simulink model "Design and Analysis of Fuel Cell Vehicle-to-Grid System"  (R2024b)
settings: Solver=VariableStepAuto  StartTime=0.0  StopTime=5  RelTol=1e-3
values from neighbouring files (symbols this model uses):
  Afc = 232.0    (= 232)    [rlpar_1.m]
  F = 96485    [rlpar_1.m]
  K1 = 7.034e-3    (= 0.007034)    [rlpar_1.m]
  K2 = 7.036e-3    (= 0.007036)    [rlpar_1.m]
  N = 35    [rlpar_1.m]
  Pop = 101325    [rlpar_1.m]
  R = 8.314    [rlpar_1.m]
  T = 338.5    [rlpar_1.m]
  Ts = 4e-6    (= 4e-06)    [rlpar_1.m]
  Va = 6.495    [rlpar_1.m]
  YH2 = 0.99    [rlpar_1.m]
  YO2 = 0.21    [rlpar_1.m]
undefined symbols (not defined in the file or in its folder): ln
libraries: powerlib_extras x14, spsSeriesRLCBranchLib x9, spsCurrentMeasurementLib x6, spsIGBTLib x5, spsVoltageMeasurementLib x4, spsControlledVoltageSourceLib x2, spsACVoltageSourceLib x1, spsDCVoltageSourceLib x1, spsDiodeLib x1, spsGroundLib x1, slpidlib x1, spsPWMGeneratorDCDCLib x1
settings Model: Creator=Ashish  LastModifiedBy=Ashish

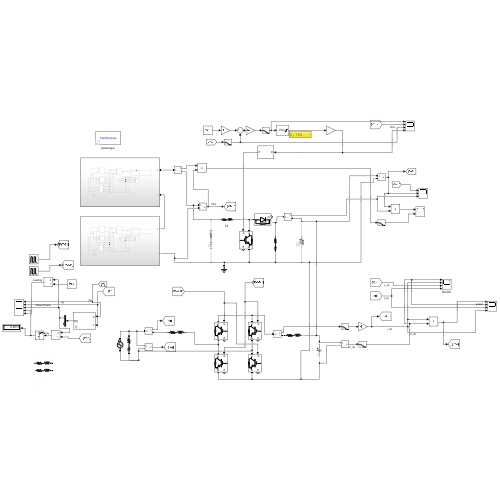
[thumbnail: Simulink's stored preview of the top-level diagram]
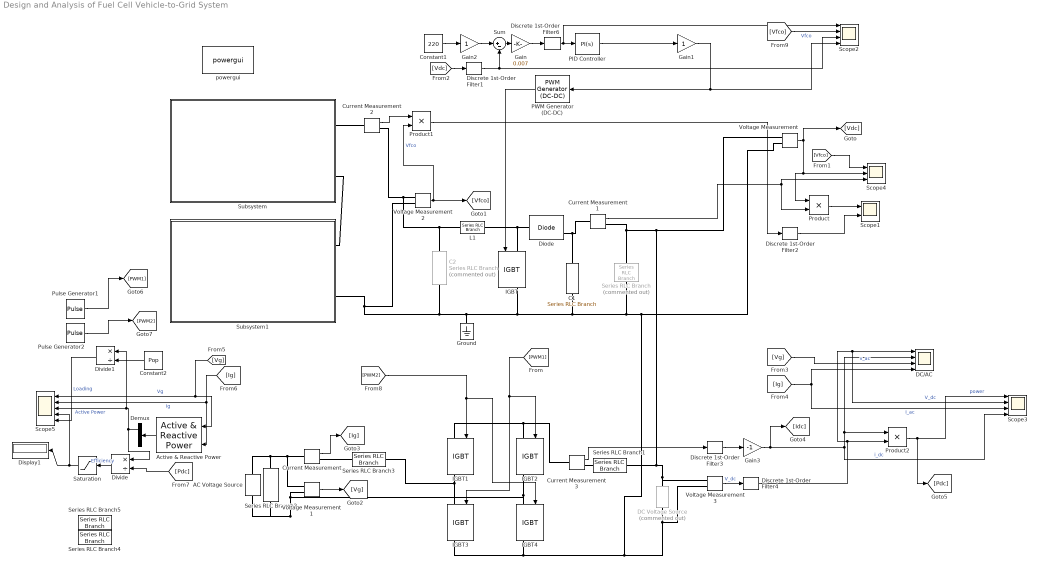
== system Design and Analysis of Fuel Cell Vehicle-to-Grid System ==
  AC Voltage Source : spsACVoltageSourceLib/AC Voltage Source  Amplitude=381  Phase=0  Frequency=50  SampleTime=0  Measurements=None  BusType=swing  Pref=10e3  Qref=0  Qmin=-inf  Qmax=+inf
  Active & Reactive Power : powerlib_extras/Measurements/Active & Reactive Power  f1=50
  C1 : spsSeriesRLCBranchLib/Series RLC Branch  LConnTagsString=__new0  RConnTagsString=__new0  BranchType=RC  Resistance=0.0001  Inductance=1.0  SetiL0=off  InitialCurrent=0  Capacitance=1e-4  Setx0=on  InitialVoltage=0  Measurements=Branch voltage
  C2 : spsSeriesRLCBranchLib/Series RLC Branch  Commented=on  LConnTagsString=__new0  RConnTagsString=__new0  BranchType=RC  Resistance=1.0  Inductance=1.0  SetiL0=off  InitialCurrent=0  Capacitance=1e-1  Setx0=off  InitialVoltage=600  Measurements=Branch voltage
  Constant1 : Constant  Value=220
  Constant2 : Constant  Value=Pop
  Current Measurement{,1..3} (4 alike) : spsCurrentMeasurementLib/Current Measurement  PhasorSimulation=off  OutputType=Complex  PSBequivalent=0
  DC Voltage Source : spsDCVoltageSourceLib/DC Voltage Source  Commented=on  Amplitude=220  Measurements=None
  DC/AC : Scope  NumInputPorts=4
  Demux : Demux  Outputs=2
  Diode : spsDiodeLib/Diode  Ron=0.001  Lon=0  Vf=0.8  IC=0  UseSnubber=off  Rs=500  Cs=250e-9  Measurements=on
  Discrete 1st-Order Filter{1..4,6} (5 alike) : powerlib_extras/Discrete  Control Blocks/Discrete 1st-Order Filter  FilterType=Lowpass  Tc=12e-3  Ts=Ts  Initialize=off  Vac_Init=[0.8 -25 60]  Vdc_Init=-0.4  PlotResponse=off  param1=[1 500 0.1]
  Display1 : Display
  Divide : Product  Inputs=*/
  Divide1 : Product  Inputs=*/
  Gain : Gain  Gain=0.007
  Gain1 : Gain
  Gain2 : Gain
  Gain3 : Gain  Gain=-1
  Ground : spsGroundLib/Ground  LConnTagsString=a
  IGBT{,1..4} (5 alike) : spsIGBTLib/IGBT  Ron=0.001  Lon=0  Vf=1  Tf=1e-6  Tt=2e-6  IC=0  Rs=1e5  Cs=inf  Measurements=on
  L1 : spsSeriesRLCBranchLib/Series RLC Branch  LConnTagsString=__new0  RConnTagsString=__new0  BranchType=RL  Resistance=0.001  Inductance=1e-3  SetiL0=off  InitialCurrent=2  Capacitance=1e-6  Setx0=off  InitialVoltage=0  Measurements=None
  PID Controller : slpidlib/PID Controller  Controller=PI  Form=Parallel  TimeDomain=Continuous-time  UseExternalTs=off  SampleTime=-1  IntegratorMethod=Forward Euler  FilterMethod=Forward Euler  ControllerParametersSource=internal  P=0.6  I=8  UseKiTs=off  D=0  UseExternalDerivativeSource=off  N=100  UseFilter=on  TunerSelectOption=Transfer Function Based (PID Tuner App)  InitialConditionSource=internal  InitialConditionForIntegrator=0.1  InitialConditionForFilter=0  DifferentiatorICPrevScaledInput=0  ExternalReset=none  TrackingMode=off  Kt=1  LimitOutput=on  SatLimitsSource=internal  UpperSaturationLimit=0.99  LowerSaturationLimit=0.1  LinearizeAsGain=on  AntiWindupMode=none  Kb=1  LimitIntegrator=off  UpperIntegratorSaturationLimit=inf  LowerIntegratorSaturationLimit=-inf  POutMin=[]  POutMax=[]  IOutMin=[]  IOutMax=[]  DOutMin=[]  DOutMax=[]  NOutMin=[]  NOutMax=[]  SumOutMin=[]  SumOutMax=[]  SaturationOutMin=[]  SaturationOutMax=[]  PParamMin=[]  PParamMax=[]  IParamMin=[]  IParamMax=[]  DParamMin=[]  DParamMax=[]  NParamMin=[]  NParamMax=[]  KbParamMin=[]  KbParamMax=[]  KtParamMin=[]  KtParamMax=[]  KbOutMin=[]  KbOutMax=[]  KtOutMin=[]  KtOutMax=[]  IntegratorOutMin=[]  IntegratorOutMax=[]  FilterOutMin=[]  FilterOutMax=[]  SumI1OutMin=[]  SumI1OutMax=[]  SumI2OutMin=[]  SumI2OutMax=[]  SumI3OutMin=[]  SumI3OutMax=[]  SumI4OutMin=[]  SumI4OutMax=[]  SumDOutMin=[]  SumDOutMax=[]  DifferentiatorOutMin=[]  DifferentiatorOutMax=[]  FilterDiffOutCoefMin=[]  FilterDiffOutCoefMax=[]  ReciprocalOutMin=[]  ReciprocalOutMax=[]  SumDenOutMin=[]  SumDenOutMax=[]  SumNumOutMin=[]  SumNumOutMax=[]  DivideOutMin=[]  DivideOutMax=[]  UdiffTsProdOutMin=[]  UdiffTsProdOutMax=[]  NTsProdOutMin=[]  NTsProdOutMax=[]  UintegralTsProdOutMin=[]  UintegralTsProdOutMax=[]  UngainTsProdOutMin=[]  UngainTsProdOutMax=[]  ClampingZeroOutDataTypeStr=Inherit: Inherit via back propagation  ClampingZeroOutMin=[]  ClampingZeroOutMax=[]  FilterDenConstantOutDataTypeStr=Inherit: Inherit via back propagation  FilterDenConstantOutMin=[]  FilterDenConstantOutMax=[]  PCopyOutDataTypeStr=Inherit: Inherit via back propagation  PCopyOutMin=[]  PCopyOutMax=[]  NCopyOutDataTypeStr=Inherit: Inherit via back propagation  NCopyOutMin=[]  NCopyOutMax=[]  IntegratorContinuousStateAttributes=''  IntegratorStateMustResolveToSignalObject=off  IntegratorRTWStateStorageClass=Auto  FilterContinuousStateAttributes=''  FilterStateMustResolveToSignalObject=off  FilterRTWStateStorageClass=Auto  ParallelPVariant=InternalParameters  IdealPVariant=Disabled  IVariant=InternalParameters  DVariant=Disabled  IntegratorVariant=Continuous  SatVariant=Enabled  AWVariant=Passthrough  PCopyVariant=Disabled  TRVariant=Disabled  FdbkBlocksVariant=Forward  IdealPFdbkVariant=Disabled  SatFdbkVariant=Disabled  DerivativeFilterVariant=Disabled  NVariant=Disabled  NCopyVariant=Disabled_SignalSpec  FilterICVariant=Disabled  IntegratorICVariant=InternalICs  ExternalResetVariant=Disabled  TRSumVariant=Passthrough  SumFdbkVariant=Disabled  SumVariant=Sum_PI  TsampFilterVariant=InternalTs  TsampNgainVariant=Passthrough  TsampIntegralVariant=Disabled_SignalSpec  ExternalSaturationOutDataTypeStr=Inherit: Same as second input  DerivativeSourceVariant=Disabled  PreIntVariant=InternalPreInt
  PWM Generator (DC-DC) : spsPWMGeneratorDCDCLib/PWM Generator (DC-DC)  Fsw=5000  Ts=0
  Product : Product
  Product1 : Product
  Product2 : Product
  Pulse Generator1 : DiscretePulseGenerator  PulseType=Time based  Period=1/50  PulseWidth=50  PhaseDelay=11/12/50
  Pulse Generator2 : DiscretePulseGenerator  PulseType=Time based  Period=1/50  PulseWidth=50  PhaseDelay=5/12/50
  Saturation : Saturate  UpperLimit=1  LowerLimit=0
  Scope1 : Scope  NumInputPorts=2
  Scope2 : Scope  NumInputPorts=4
  Scope3 : Scope  NumInputPorts=4
  Scope4 : Scope  NumInputPorts=3
  Scope5 : Scope  NumInputPorts=5
  Series RLC Branch : spsSeriesRLCBranchLib/Series RLC Branch  Commented=on  LConnTagsString=__new0  RConnTagsString=__new0  BranchType=R  Resistance=100  Inductance=1e-3  SetiL0=off  InitialCurrent=0  Capacitance=1e-6  Setx0=off  InitialVoltage=0  Measurements=None
  Series RLC Branch1 : spsSeriesRLCBranchLib/Series RLC Branch  LConnTagsString=__new0  RConnTagsString=__new0  BranchType=RL  Resistance=0.01  Inductance=1  SetiL0=on  InitialCurrent=20  Capacitance=1e-6  Setx0=off  InitialVoltage=0  Measurements=None
  Series RLC Branch2 : spsSeriesRLCBranchLib/Series RLC Branch  LConnTagsString=__new0  RConnTagsString=__new0  BranchType=RC  Resistance=0.00001  Inductance=100  SetiL0=on  InitialCurrent=-1  Capacitance=1e-2  Setx0=off  InitialVoltage=0  Measurements=None
  Series RLC Branch3 : spsSeriesRLCBranchLib/Series RLC Branch  LConnTagsString=__new0  RConnTagsString=__new0  BranchType=RL  Resistance=6  Inductance=0.00001  SetiL0=on  InitialCurrent=0  Capacitance=1e-6  Setx0=off  InitialVoltage=0  Measurements=None
  Series RLC Branch4 : spsSeriesRLCBranchLib/Series RLC Branch  LConnTagsString=__new0  RConnTagsString=__new0  BranchType=RL  Resistance=10  Inductance=1  SetiL0=on  InitialCurrent=20  Capacitance=1e-6  Setx0=off  InitialVoltage=0  Measurements=None
  Series RLC Branch5 : spsSeriesRLCBranchLib/Series RLC Branch  LConnTagsString=__new0  RConnTagsString=__new0  BranchType=RL  Resistance=10  Inductance=0.00001  SetiL0=on  InitialCurrent=0  Capacitance=1e-6  Setx0=off  InitialVoltage=0  Measurements=None
  Subsystem : Subsystem
  Subsystem1 : Subsystem
  Sum : Sum  Inputs=|+-
  Voltage Measurement{,1..3} (4 alike) : spsVoltageMeasurementLib/Voltage Measurement  PhasorSimulation=off  OutputType=Complex  PSBequivalent=0
  powergui : sps_lib/powergui  Priority=1  SimulationMode=Continuous  SampleTime=Ts  frequency=60  Iterations=50  frequencyindice=0  Pbase=100e6  ErrMax=1e-4  UnitsV=kV  UnitsW=MW  buscounter=0  FunctionMessages=off  echomessages=off  EnableUseOfTLC=off  CurrentSourceSwitches=off  DisableSnubberDevices=off  DisableRonSwitches=off  DisableVfSwitches=off  DisplayEquations=off  AutomaticDiscreteSolvers=off  SolverType=Tustin/Backward Euler (TBE)  Interpol=off  ExternalGateDelay=off  methode=off  Ts=100  x0status=blocks  SPID=off  SwTol=0  HookPort=off  NonlinearTolerance=1e-4  nMaxIteration=100  ContinueOnMaxIteration=off  RestoreLinks=warning  ResistiveCurrentMeasurement=off  Frange=[0:2:500]  Ylog=off  Xlog=on  ShowGrid=off  save=off  variable=ZData  structure=0  ZoomFFT=off  StartTime=0.0  cycles=1  DisplayStyle=1  fundamental=60  FreqAxis=off  MaxFrequency=1000  frequencyindicesteady=1  RmsSteady=1  display=off
  wires:
  Discrete 1st-Order Filter3/1 -> Gain3/1
  Current Measurement2/1 -> Product1/1
  [Vdc] -> Discrete 1st-Order Filter1/1
  Constant1/1 -> Gain2/1
  Current Measurement1/1 -> Scope4/3, Product/2
  Pulse Generator1/1 -> [PWM1]
  Gain2/1 -> Sum/1
  Product2/1 -> Scope3/1, [Pdc]  "power"
  Product/1 -> Scope1/1
  Discrete 1st-Order Filter2/1 -> Scope1/2
  Discrete 1st-Order Filter6/1 -> Scope2/1, PID Controller/1
  Voltage Measurement2/1 -> Product1/2, [Vfco]  "Vfco"
  Gain1/1 -> PWM Generator (DC-DC)/1, Scope2/4
  Voltage Measurement3/1 -> Discrete 1st-Order Filter4/1  "V_dc"
  Discrete 1st-Order Filter1/1 -> Sum/2, Scope2/3
  Voltage Measurement/1 -> [Vdc], Scope4/2, Product/1
  PID Controller/1 -> Gain1/1
  Product1/1 -> Discrete 1st-Order Filter2/1
  Discrete 1st-Order Filter4/1 -> Scope3/2, DC/AC/1, Product2/2  "V_dc"
  Voltage Measurement1/1 -> [Vg]
  Gain3/1 -> [Idc], DC/AC/2, Product2/1, Scope3/4  "i_dc"
  [Ig] -> Scope3/3, DC/AC/4  "I_ac"
  Current Measurement3/1 -> Discrete 1st-Order Filter3/1
  PWM Generator (DC-DC)/1 -> IGBT/1
  Current Measurement/1 -> [Ig]
  [Vfco] -> Scope4/1
  [Vg] -> DC/AC/3  "v_ac"
  Gain/1 -> Discrete 1st-Order Filter6/1
  Sum/1 -> Gain/1
  [Vg] -> Active & Reactive Power/1, Scope5/1  "Vg"
  [Ig] -> Active & Reactive Power/2, Scope5/2  "Ig"
  Active & Reactive Power/1 -> Demux/1
  Demux/1 -> Divide/1, Divide1/1, Scope5/3  "Active Power"
  Divide/1 -> Saturation/1  "Efficiency"
  [Pdc] -> Divide/2
  Divide1/1 -> Scope5/5  "Loading"
  Constant2/1 -> Divide1/2
  Saturation/1 -> Display1/1, Scope5/4
  [PWM1] -> IGBT3/1, IGBT2/1
  [PWM2] -> IGBT4/1, IGBT1/1
  Pulse Generator2/1 -> [PWM2]
  [Vfco] -> Scope2/2  "Vfco"
  connections:
  Voltage Measurement3/LConn2 -- Series RLC Branch/RConn1 -- C1/RConn1 -- Ground/LConn1 -- Subsystem1/RConn2 -- Voltage Measurement2/LConn2 -- C2/RConn1 -- IGBT/RConn1 -- Voltage Measurement/LConn2 -- IGBT3/RConn1 -- IGBT4/RConn1 -- DC Voltage Source/LConn1
  Diode/LConn1 -- IGBT/LConn1 -- L1/RConn1
  Series RLC Branch2/RConn1 -- IGBT4/LConn1 -- IGBT2/RConn1 -- Voltage Measurement1/LConn2 -- AC Voltage Source/LConn1
  Current Measurement1/RConn1 -- Voltage Measurement3/LConn1 -- DC Voltage Source/RConn1 -- Series RLC Branch1/RConn1 -- Voltage Measurement/LConn1 -- Series RLC Branch/LConn1
  IGBT1/LConn1 -- IGBT2/LConn1 -- Current Measurement3/LConn1
  Current Measurement2/RConn1 -- C2/LConn1 -- L1/LConn1 -- Voltage Measurement2/LConn1
  Voltage Measurement1/LConn1 -- Current Measurement/LConn1 -- AC Voltage Source/RConn1 -- Series RLC Branch2/LConn1
  IGBT3/LConn1 -- IGBT1/RConn1 -- Series RLC Branch3/RConn1
  C1/LConn1 -- Current Measurement1/LConn1 -- Diode/RConn1
  Current Measurement2/LConn1 -- Subsystem/RConn1
  Current Measurement3/RConn1 -- Series RLC Branch1/LConn1
  Current Measurement/RConn1 -- Series RLC Branch3/LConn1
  Subsystem/RConn2 -- Subsystem1/RConn1

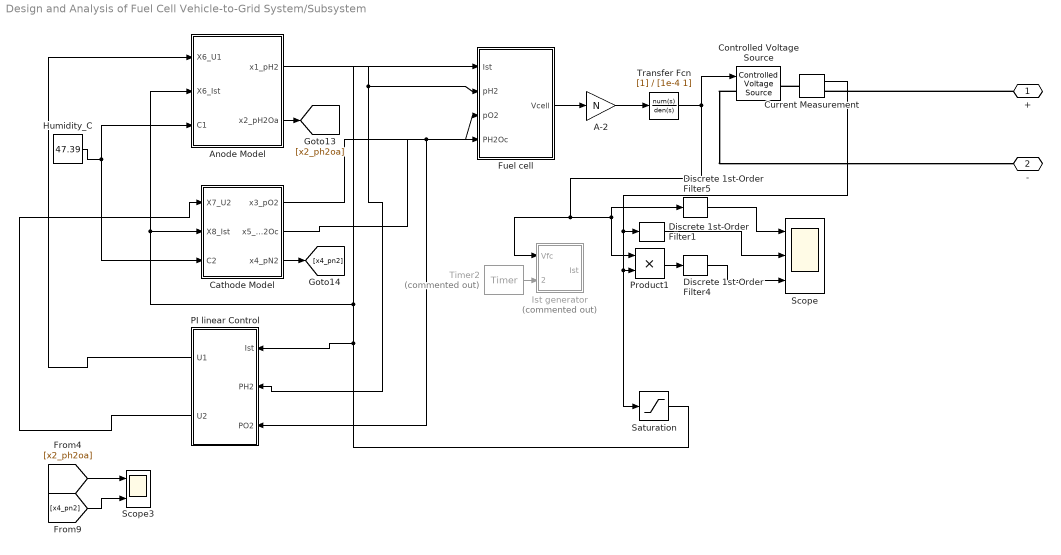
== system Design and Analysis of Fuel Cell Vehicle-to-Grid System/Subsystem ==
  A-2 : Gain  Gain=N  SaturateOnIntegerOverflow=on  OutDataTypeStr=Inherit: Same as input  ParamDataTypeStr=Inherit: Same as input
  Anode Model : Subsystem
  Cathode Model : Subsystem
  Controlled Voltage Source : spsControlledVoltageSourceLib/Controlled Voltage Source  Initialize=on  Source_Type=DC  Amplitude=0  Phase=0  Frequency=0  Measurements=None
  Current Measurement : spsCurrentMeasurementLib/Current Measurement  PhasorSimulation=off  OutputType=Complex  PSBequivalent=0
  Discrete 1st-Order Filter1 : powerlib_extras/Discrete  Control Blocks/Discrete 1st-Order Filter  FilterType=Lowpass  Tc=12e-3  Ts=Ts  Initialize=off  Vac_Init=[0.8 -25 60]  Vdc_Init=-0.4  PlotResponse=off  param1=[1 500 0.1]
  Discrete 1st-Order Filter4 : powerlib_extras/Discrete  Control Blocks/Discrete 1st-Order Filter  FilterType=Lowpass  Tc=12e-3  Ts=Ts  Initialize=off  Vac_Init=[0.8 -25 60]  Vdc_Init=-0.4  PlotResponse=off  param1=[1 500 0.1]
  Discrete 1st-Order Filter5 : powerlib_extras/Discrete  Control Blocks/Discrete 1st-Order Filter  FilterType=Lowpass  Tc=12e-3  Ts=Ts  Initialize=off  Vac_Init=[0.8 -25 60]  Vdc_Init=-0.4  PlotResponse=off  param1=[1 500 0.1]
  Fuel cell : Subsystem
  Humidity_C : Constant  Value=47.39
  Ist generator : Subsystem  Commented=on
  "PI linear Control " : Subsystem
  Product1 : Product
  Saturation : Saturate  UpperLimit=10000  LowerLimit=0
  Scope : Scope  NumInputPorts=3
  Scope3 : Scope  NumInputPorts=2
  Timer2 : powerlib_extras/Control  Blocks/Timer  Commented=on  t=[ 0 1.50 2.00 2.50 3.00 3.50 4.00 4.50 5.0 5.5]  e="[1  0.6  0.3 0.175 0.3 1 2.5 5 1 5 ]"
  Transfer Fcn : TransferFcn  Denominator=[1e-4 1]
  + : PMIOPort  Side=Right
  - : PMIOPort  Port=2  Side=Right
  wires:
  [x2_ph2oa] -> Scope3/1
  Discrete 1st-Order Filter5/1 -> Scope/1
  Transfer Fcn/1 -> Discrete 1st-Order Filter5/1, Product1/1, Ist generator/1(Vfc), Controlled Voltage Source/1
  Fuel cell/1("Vcell ") -> A-2/1
  Discrete 1st-Order Filter1/1 -> Scope/2
  Anode Model/2(x2_pH2Oa) -> [x2_ph2oa]
  Saturation/1 -> Fuel cell/1(Ist), Anode Model/2(X6_Ist), Cathode Model/2(X8_Ist), "PI linear Control "/1(Ist)
  Anode Model/1(x1_pH2) -> Fuel cell/2(pH2), "PI linear Control "/2(PH2)
  Product1/1 -> Discrete 1st-Order Filter4/1
  Cathode Model/1(x3_pO2) -> Fuel cell/3(pO2), "PI linear Control "/3(PO2)
  Current Measurement/1 -> Saturation/1, Product1/2, Discrete 1st-Order Filter1/1
  [x4_pn2] -> Scope3/2
  Humidity_C/1 -> Cathode Model/3(C2), Anode Model/3(C1)
  "PI linear Control "/1("U1 ") -> Anode Model/1(X6_U1)
  A-2/1 -> Transfer Fcn/1
  Discrete 1st-Order Filter4/1 -> Scope/3
  Cathode Model/3(x4_pN2) -> [x4_pn2]
  Cathode Model/2(x5_pH2Oc) -> Fuel cell/4(PH2Oc)
  Timer2/1 -> Ist generator/2(Rload)
  "PI linear Control "/2(U2) -> Cathode Model/1(X7_U2)
  connections:
  Current Measurement/LConn1 -- Controlled Voltage Source/RConn1
  +/RConn1 -- Current Measurement/RConn1
  Controlled Voltage Source/LConn1 -- -/RConn1

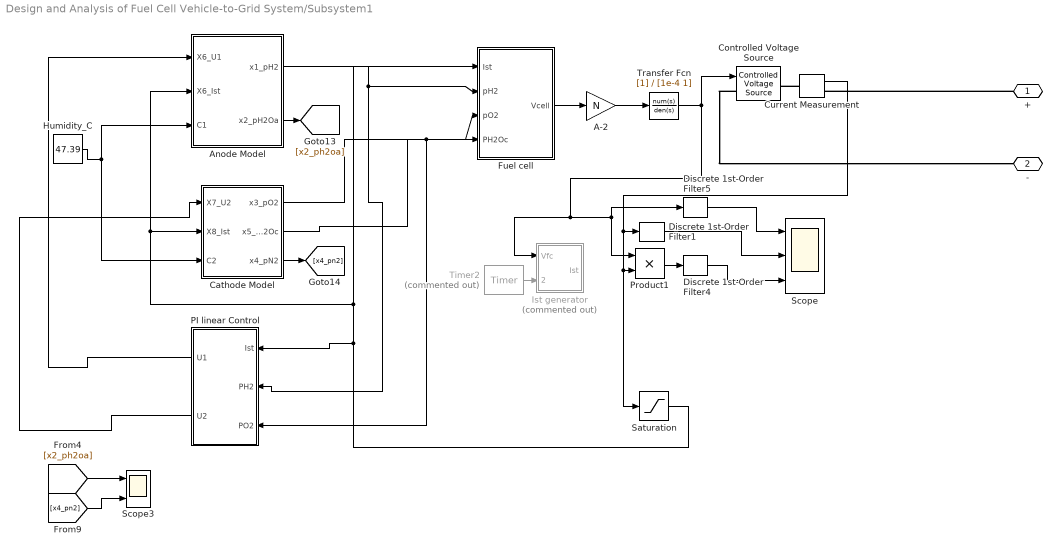
== system Design and Analysis of Fuel Cell Vehicle-to-Grid System/Subsystem1 ==
  A-2 : Gain  Gain=N  SaturateOnIntegerOverflow=on  OutDataTypeStr=Inherit: Same as input  ParamDataTypeStr=Inherit: Same as input
  Anode Model : Subsystem
  Cathode Model : Subsystem
  Controlled Voltage Source : spsControlledVoltageSourceLib/Controlled Voltage Source  Initialize=on  Source_Type=DC  Amplitude=0  Phase=0  Frequency=0  Measurements=None
  Current Measurement : spsCurrentMeasurementLib/Current Measurement  PhasorSimulation=off  OutputType=Complex  PSBequivalent=0
  Discrete 1st-Order Filter1 : powerlib_extras/Discrete  Control Blocks/Discrete 1st-Order Filter  FilterType=Lowpass  Tc=12e-3  Ts=Ts  Initialize=off  Vac_Init=[0.8 -25 60]  Vdc_Init=-0.4  PlotResponse=off  param1=[1 500 0.1]
  Discrete 1st-Order Filter4 : powerlib_extras/Discrete  Control Blocks/Discrete 1st-Order Filter  FilterType=Lowpass  Tc=12e-3  Ts=Ts  Initialize=off  Vac_Init=[0.8 -25 60]  Vdc_Init=-0.4  PlotResponse=off  param1=[1 500 0.1]
  Discrete 1st-Order Filter5 : powerlib_extras/Discrete  Control Blocks/Discrete 1st-Order Filter  FilterType=Lowpass  Tc=12e-3  Ts=Ts  Initialize=off  Vac_Init=[0.8 -25 60]  Vdc_Init=-0.4  PlotResponse=off  param1=[1 500 0.1]
  Fuel cell : Subsystem
  Humidity_C : Constant  Value=47.39
  Ist generator : Subsystem  Commented=on
  "PI linear Control " : Subsystem
  Product1 : Product
  Saturation : Saturate  UpperLimit=10000  LowerLimit=0
  Scope : Scope  NumInputPorts=3
  Scope3 : Scope  NumInputPorts=2
  Timer2 : powerlib_extras/Control  Blocks/Timer  Commented=on  t=[ 0 1.50 2.00 2.50 3.00 3.50 4.00 4.50 5.0 5.5]  e="[1  0.6  0.3 0.175 0.3 1 2.5 5 1 5 ]"
  Transfer Fcn : TransferFcn  Denominator=[1e-4 1]
  + : PMIOPort  Side=Right
  - : PMIOPort  Port=2  Side=Right
  wires:
  "PI linear Control "/2(U2) -> Cathode Model/1(X7_U2)
  Timer2/1 -> Ist generator/2(Rload)
  Cathode Model/2(x5_pH2Oc) -> Fuel cell/4(PH2Oc)
  Cathode Model/3(x4_pN2) -> [x4_pn2]
  Discrete 1st-Order Filter4/1 -> Scope/3
  A-2/1 -> Transfer Fcn/1
  "PI linear Control "/1("U1 ") -> Anode Model/1(X6_U1)
  Humidity_C/1 -> Anode Model/3(C1), Cathode Model/3(C2)
  [x4_pn2] -> Scope3/2
  Current Measurement/1 -> Discrete 1st-Order Filter1/1, Product1/2, Saturation/1
  Cathode Model/1(x3_pO2) -> "PI linear Control "/3(PO2), Fuel cell/3(pO2)
  Product1/1 -> Discrete 1st-Order Filter4/1
  Anode Model/1(x1_pH2) -> "PI linear Control "/2(PH2), Fuel cell/2(pH2)
  Saturation/1 -> "PI linear Control "/1(Ist), Cathode Model/2(X8_Ist), Anode Model/2(X6_Ist), Fuel cell/1(Ist)
  Anode Model/2(x2_pH2Oa) -> [x2_ph2oa]
  Discrete 1st-Order Filter1/1 -> Scope/2
  Fuel cell/1("Vcell ") -> A-2/1
  Transfer Fcn/1 -> Controlled Voltage Source/1, Ist generator/1(Vfc), Product1/1, Discrete 1st-Order Filter5/1
  Discrete 1st-Order Filter5/1 -> Scope/1
  [x2_ph2oa] -> Scope3/1
  connections:
  Controlled Voltage Source/LConn1 -- -/RConn1
  +/RConn1 -- Current Measurement/RConn1
  Current Measurement/LConn1 -- Controlled Voltage Source/RConn1

== system Design and Analysis of Fuel Cell Vehicle-to-Grid System/Subsystem/Anode Model ==
  X6_U1 : Inport
  X6_Ist : Inport  Port=2
  C1 : Inport  Port=3
  Abs : Abs
  Abs1 : Abs
  Hydrogen Model : Subsystem
  Saturation1 : Saturate  UpperLimit=100  LowerLimit=0
  Saturation2 : Saturate  UpperLimit=100  LowerLimit=0
  "Water Model " : Subsystem
  x1_pH2 : Outport
  x2_pH2Oa : Outport  Port=2
  wires:
  X6_U1/1 -> Hydrogen Model/1(x6), "Water Model "/1(x6)
  X6_Ist/1 -> Hydrogen Model/2(x8)
  Hydrogen Model/1(pH2_x1) -> Abs/1
  Abs/1 -> Saturation2/1
  Abs1/1 -> Saturation1/1
  Saturation1/1 -> Hydrogen Model/3(pH20_a_x2), x2_pH2Oa/1
  "Water Model "/1(pH2O_a_x2) -> Abs1/1
  C1/1 -> "Water Model "/3(C1)
  Saturation2/1 -> x1_pH2/1, "Water Model "/2(pH2_x1)

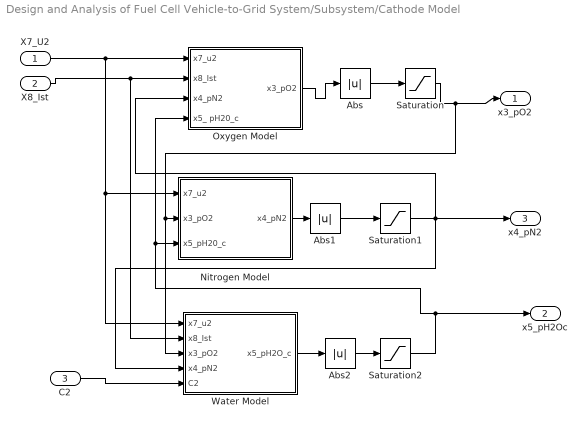
== system Design and Analysis of Fuel Cell Vehicle-to-Grid System/Subsystem/Cathode Model ==
  X7_U2 : Inport
  X8_Ist : Inport  Port=2
  C2 : Inport  Port=3
  Abs : Abs
  Abs1 : Abs
  Abs2 : Abs
  Nitrogen Model : Subsystem
  Oxygen Model : Subsystem
  Saturation : Saturate  UpperLimit=100  LowerLimit=0
  Saturation1 : Saturate  UpperLimit=100  LowerLimit=0
  Saturation2 : Saturate  UpperLimit=100  LowerLimit=0.001
  "Water Model " : Subsystem
  x3_pO2 : Outport
  x5_pH2Oc : Outport  Port=2
  x4_pN2 : Outport  Port=3
  wires:
  X7_U2/1 -> "Water Model "/1(x7_u2), Nitrogen Model/1(x7_u2), Oxygen Model/1(x7_u2)
  Oxygen Model/1(x3_pO2) -> Abs/1
  "Water Model "/1(x5_pH2O_c) -> Abs2/1
  X8_Ist/1 -> "Water Model "/2(x8_Ist), Oxygen Model/2(x8_Ist)
  Nitrogen Model/1(x4_pN2) -> Abs1/1
  C2/1 -> "Water Model "/5(C2)
  Abs1/1 -> Saturation1/1
  Abs/1 -> Saturation/1
  Abs2/1 -> Saturation2/1
  Saturation/1 -> x3_pO2/1, "Water Model "/3(x3_pO2), Nitrogen Model/2(x3_pO2)
  Saturation1/1 -> Oxygen Model/3(x4_pN2), x4_pN2/1, "Water Model "/4(x4_pN2)
  Saturation2/1 -> Oxygen Model/4(x5_ pH20_c), Nitrogen Model/3(x5_pH20_c), x5_pH2Oc/1

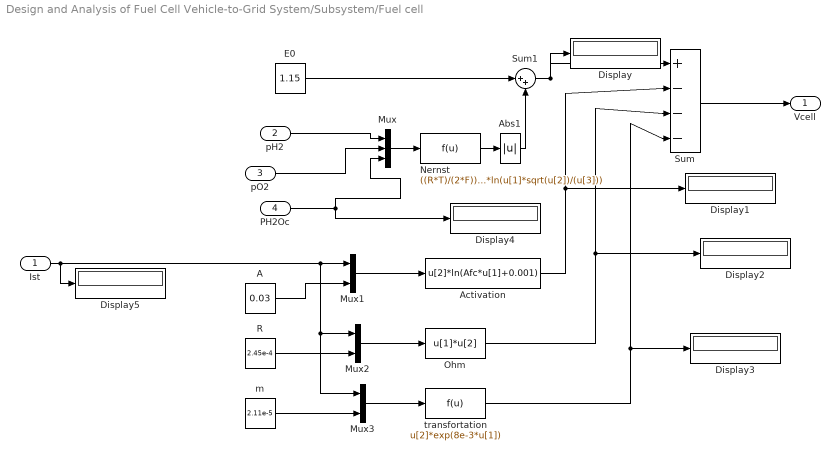
== system Design and Analysis of Fuel Cell Vehicle-to-Grid System/Subsystem/Fuel cell ==
  Ist : Inport
  pH2 : Inport  Port=2
  pO2 : Inport  Port=3
  PH2Oc : Inport  Port=4
  A : Constant  Value=0.03
  Abs1 : Abs
  Activation : Fcn  Expr=u[2]*ln(Afc*u[1]+0.001)
  Display{,1..5} (6 alike) : Display
  E0 : Constant  Value=1.15
  Mux : Mux  Inputs=3
  Mux1 : Mux  Inputs=2
  Mux2 : Mux  Inputs=2
  Mux3 : Mux  Inputs=2
  Nernst : Fcn  Expr=((R*T)/(2*F))*ln(u[1]*sqrt(u[2])/(u[3]))
  Ohm : Fcn  Expr=u[1]*u[2]
  R : Constant  Value=2.45e-4
  Sum : Sum  Inputs=|+---|  SaturateOnIntegerOverflow=on
  Sum1 : Sum  Inputs=|++  SaturateOnIntegerOverflow=on
  m : Constant  Value=2.11e-5
  transfortation : Fcn  Expr=u[2]*exp(8e-3*u[1])
  "Vcell " : Outport
  wires:
  pH2/1 -> Mux/1
  PH2Oc/1 -> Display4/1, Mux/3
  Mux/1 -> Nernst/1
  E0/1 -> Sum1/1
  Nernst/1 -> Abs1/1
  Sum1/1 -> Sum/1, Display/1
  Ist/1 -> Display5/1, Mux3/1, Mux2/1, Mux1/1
  Mux1/1 -> Activation/1
  A/1 -> Mux1/2
  Activation/1 -> Sum/2, Display1/1
  R/1 -> Mux2/2
  Mux2/1 -> Ohm/1
  Ohm/1 -> Sum/3, Display2/1
  m/1 -> Mux3/2
  Mux3/1 -> transfortation/1
  transfortation/1 -> Sum/4, Display3/1
  Sum/1 -> "Vcell "/1
  pO2/1 -> Mux/2
  Abs1/1 -> Sum1/2

== system Design and Analysis of Fuel Cell Vehicle-to-Grid System/Subsystem/Ist generator ==
  Vfc : Inport
  Rload : Inport  Port=2
  Constat : Constant  Value=0
  Fcn : Fcn  Expr=u[1]/u[2]
  Mux : Mux  Inputs=2
  Saturation : Saturate  UpperLimit=10000  LowerLimit=0
  Sum : Sum  Inputs=|++  SaturateOnIntegerOverflow=on
  Ist : Outport
  wires:
  Mux/1 -> Fcn/1
  Fcn/1 -> Saturation/1
  Saturation/1 -> Sum/1
  Constat/1 -> Sum/2
  Vfc/1 -> Mux/1
  Sum/1 -> Ist/1
  Rload/1 -> Mux/2

== system Design and Analysis of Fuel Cell Vehicle-to-Grid System/Subsystem/PI linear Control  ==
  Ist : Inport
  PH2 : Inport  Port=2
  PO2 : Inport  Port=3
  Display2 : Display
  Linear PI  v1 : Subsystem
  Linear PI  v2 : Subsystem
  limiter : Saturate  UpperLimit=1000  LowerLimit=0  ZeroCross=off
  limiter1 : Saturate  UpperLimit=1000  LowerLimit=0  ZeroCross=off
  "U1 " : Outport
  U2 : Outport  Port=2
  wires:
  Linear PI  v1/1("v2 ") -> limiter/1
  Ist/1 -> Linear PI  v2/2(Ist), Linear PI  v1/2(Ist)
  PH2/1 -> Linear PI  v1/1(pO2)
  Linear PI  v2/1("v2 ") -> limiter1/1
  PO2/1 -> Linear PI  v2/1(pO2)
  limiter/1 -> Display2/1, "U1 "/1
  limiter1/1 -> U2/1

== system Design and Analysis of Fuel Cell Vehicle-to-Grid System/Subsystem1/Anode Model ==
  X6_U1 : Inport
  X6_Ist : Inport  Port=2
  C1 : Inport  Port=3
  Abs : Abs
  Abs1 : Abs
  Hydrogen Model : Subsystem
  Saturation1 : Saturate  UpperLimit=100  LowerLimit=0
  Saturation2 : Saturate  UpperLimit=100  LowerLimit=0
  "Water Model " : Subsystem
  x1_pH2 : Outport
  x2_pH2Oa : Outport  Port=2
  wires:
  Saturation2/1 -> "Water Model "/2(pH2_x1), x1_pH2/1
  C1/1 -> "Water Model "/3(C1)
  "Water Model "/1(pH2O_a_x2) -> Abs1/1
  Saturation1/1 -> x2_pH2Oa/1, Hydrogen Model/3(pH20_a_x2)
  Abs1/1 -> Saturation1/1
  Abs/1 -> Saturation2/1
  Hydrogen Model/1(pH2_x1) -> Abs/1
  X6_Ist/1 -> Hydrogen Model/2(x8)
  X6_U1/1 -> "Water Model "/1(x6), Hydrogen Model/1(x6)

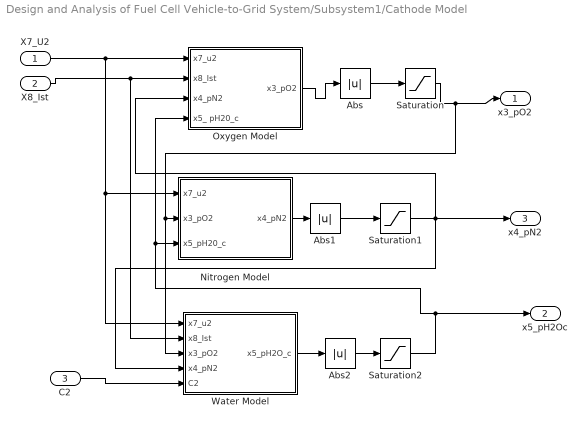
== system Design and Analysis of Fuel Cell Vehicle-to-Grid System/Subsystem1/Cathode Model ==
  X7_U2 : Inport
  X8_Ist : Inport  Port=2
  C2 : Inport  Port=3
  Abs : Abs
  Abs1 : Abs
  Abs2 : Abs
  Nitrogen Model : Subsystem
  Oxygen Model : Subsystem
  Saturation : Saturate  UpperLimit=100  LowerLimit=0
  Saturation1 : Saturate  UpperLimit=100  LowerLimit=0
  Saturation2 : Saturate  UpperLimit=100  LowerLimit=0.001
  "Water Model " : Subsystem
  x3_pO2 : Outport
  x5_pH2Oc : Outport  Port=2
  x4_pN2 : Outport  Port=3
  wires:
  Saturation2/1 -> x5_pH2Oc/1, Nitrogen Model/3(x5_pH20_c), Oxygen Model/4(x5_ pH20_c)
  Saturation1/1 -> "Water Model "/4(x4_pN2), x4_pN2/1, Oxygen Model/3(x4_pN2)
  Saturation/1 -> Nitrogen Model/2(x3_pO2), "Water Model "/3(x3_pO2), x3_pO2/1
  Abs2/1 -> Saturation2/1
  Abs/1 -> Saturation/1
  Abs1/1 -> Saturation1/1
  C2/1 -> "Water Model "/5(C2)
  Nitrogen Model/1(x4_pN2) -> Abs1/1
  X8_Ist/1 -> Oxygen Model/2(x8_Ist), "Water Model "/2(x8_Ist)
  "Water Model "/1(x5_pH2O_c) -> Abs2/1
  Oxygen Model/1(x3_pO2) -> Abs/1
  X7_U2/1 -> Oxygen Model/1(x7_u2), Nitrogen Model/1(x7_u2), "Water Model "/1(x7_u2)

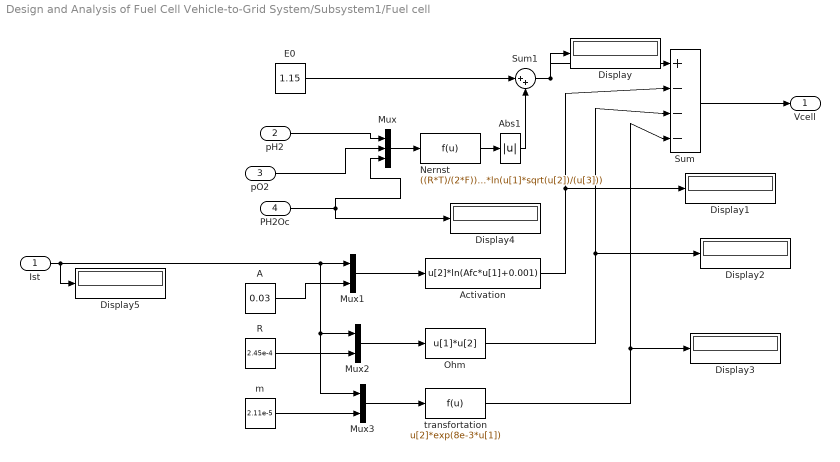
== system Design and Analysis of Fuel Cell Vehicle-to-Grid System/Subsystem1/Fuel cell ==
  Ist : Inport
  pH2 : Inport  Port=2
  pO2 : Inport  Port=3
  PH2Oc : Inport  Port=4
  A : Constant  Value=0.03
  Abs1 : Abs
  Activation : Fcn  Expr=u[2]*ln(Afc*u[1]+0.001)
  Display{,1..5} (6 alike) : Display
  E0 : Constant  Value=1.15
  Mux : Mux  Inputs=3
  Mux1 : Mux  Inputs=2
  Mux2 : Mux  Inputs=2
  Mux3 : Mux  Inputs=2
  Nernst : Fcn  Expr=((R*T)/(2*F))*ln(u[1]*sqrt(u[2])/(u[3]))
  Ohm : Fcn  Expr=u[1]*u[2]
  R : Constant  Value=2.45e-4
  Sum : Sum  Inputs=|+---|  SaturateOnIntegerOverflow=on
  Sum1 : Sum  Inputs=|++  SaturateOnIntegerOverflow=on
  m : Constant  Value=2.11e-5
  transfortation : Fcn  Expr=u[2]*exp(8e-3*u[1])
  "Vcell " : Outport
  wires:
  Abs1/1 -> Sum1/2
  pO2/1 -> Mux/2
  Sum/1 -> "Vcell "/1
  transfortation/1 -> Display3/1, Sum/4
  Mux3/1 -> transfortation/1
  m/1 -> Mux3/2
  Ohm/1 -> Display2/1, Sum/3
  Mux2/1 -> Ohm/1
  R/1 -> Mux2/2
  Activation/1 -> Display1/1, Sum/2
  A/1 -> Mux1/2
  Mux1/1 -> Activation/1
  Ist/1 -> Mux1/1, Mux2/1, Mux3/1, Display5/1
  Sum1/1 -> Display/1, Sum/1
  Nernst/1 -> Abs1/1
  E0/1 -> Sum1/1
  Mux/1 -> Nernst/1
  PH2Oc/1 -> Mux/3, Display4/1
  pH2/1 -> Mux/1

== system Design and Analysis of Fuel Cell Vehicle-to-Grid System/Subsystem1/Ist generator ==
  Vfc : Inport
  Rload : Inport  Port=2
  Constat : Constant  Value=0
  Fcn : Fcn  Expr=u[1]/u[2]
  Mux : Mux  Inputs=2
  Saturation : Saturate  UpperLimit=10000  LowerLimit=0
  Sum : Sum  Inputs=|++  SaturateOnIntegerOverflow=on
  Ist : Outport
  wires:
  Rload/1 -> Mux/2
  Sum/1 -> Ist/1
  Vfc/1 -> Mux/1
  Constat/1 -> Sum/2
  Saturation/1 -> Sum/1
  Fcn/1 -> Saturation/1
  Mux/1 -> Fcn/1

== system Design and Analysis of Fuel Cell Vehicle-to-Grid System/Subsystem1/PI linear Control  ==
  Ist : Inport
  PH2 : Inport  Port=2
  PO2 : Inport  Port=3
  Display2 : Display
  Linear PI  v1 : Subsystem
  Linear PI  v2 : Subsystem
  limiter : Saturate  UpperLimit=1000  LowerLimit=0  ZeroCross=off
  limiter1 : Saturate  UpperLimit=1000  LowerLimit=0  ZeroCross=off
  "U1 " : Outport
  U2 : Outport  Port=2
  wires:
  limiter1/1 -> U2/1
  limiter/1 -> "U1 "/1, Display2/1
  PO2/1 -> Linear PI  v2/1(pO2)
  Linear PI  v2/1("v2 ") -> limiter1/1
  PH2/1 -> Linear PI  v1/1(pO2)
  Ist/1 -> Linear PI  v1/2(Ist), Linear PI  v2/2(Ist)
  Linear PI  v1/1("v2 ") -> limiter/1

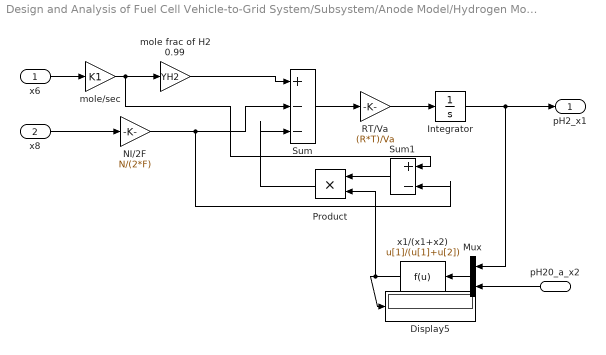
== system Design and Analysis of Fuel Cell Vehicle-to-Grid System/Subsystem/Anode Model/Hydrogen Model ==
  x6 : Inport
  x8 : Inport  Port=2
  pH20_a_x2 : Inport  Port=3
  Display5 : Display
  Integrator : Integrator  InitialCondition=1
  Mux : Mux  Inputs=2
  NI/2F : Gain  Gain=N/(2*F)  SaturateOnIntegerOverflow=on  OutDataTypeStr=Inherit: Same as input  ParamDataTypeStr=Inherit: Same as input
  Product : Product  SaturateOnIntegerOverflow=on  OutDataTypeStr=Inherit: Same as first input
  RT/Va : Gain  Gain=(R*T)/Va  SaturateOnIntegerOverflow=on  OutDataTypeStr=Inherit: Same as input  ParamDataTypeStr=Inherit: Same as input
  Sum : Sum  Inputs=|+--|  SaturateOnIntegerOverflow=on
  Sum1 : Sum  Inputs=|+-|  SaturateOnIntegerOverflow=on
  mole frac of H2 0.99 : Gain  Gain=YH2  SaturateOnIntegerOverflow=on  OutDataTypeStr=Inherit: Same as input  ParamDataTypeStr=Inherit: Same as input
  mole/sec : Gain  Gain=K1  SaturateOnIntegerOverflow=on  OutDataTypeStr=Inherit: Same as input  ParamDataTypeStr=Inherit: Same as input
  x1/(x1+x2) : Fcn  Expr=u[1]/(u[1]+u[2])
  pH2_x1 : Outport
  wires:
  mole frac of H2 0.99/1 -> Sum/1
  mole/sec/1 -> mole frac of H2 0.99/1, Sum1/1
  NI/2F/1 -> Sum/2, Sum1/2
  Sum/1 -> RT/Va/1
  RT/Va/1 -> Integrator/1
  Integrator/1 -> pH2_x1/1, Mux/1
  x6/1 -> mole/sec/1
  x8/1 -> NI/2F/1
  Sum1/1 -> Product/1
  Mux/1 -> x1/(x1+x2)/1
  pH20_a_x2/1 -> Mux/2
  x1/(x1+x2)/1 -> Product/2, Display5/1
  Product/1 -> Sum/3

== system Design and Analysis of Fuel Cell Vehicle-to-Grid System/Subsystem/Anode Model/Water Model  ==
  x6 : Inport
  pH2_x1 : Inport  Port=2
  C1 : Inport  Port=3
  C1/(x1+x2-C2) : Fcn  Expr=u[3]/(u[1]+u[2]-u[3])
  Integrator : Integrator  InitialCondition=1
  Mux : Mux  Inputs=2
  Mux1 : Mux  Inputs=3
  Product : Product  SaturateOnIntegerOverflow=on  OutDataTypeStr=Inherit: Same as first input
  Product1 : Product  SaturateOnIntegerOverflow=on  OutDataTypeStr=Inherit: Same as first input
  RT/Va : Gain  Gain=(R*T)/Va  SaturateOnIntegerOverflow=on  OutDataTypeStr=Inherit: Same as input  ParamDataTypeStr=Inherit: Same as input
  Sum : Sum  Inputs=|+-|  SaturateOnIntegerOverflow=on
  mole/sec : Gain  Gain=K1  SaturateOnIntegerOverflow=on  OutDataTypeStr=Inherit: Same as input  ParamDataTypeStr=Inherit: Same as input
  x1/(x1+x2) : Fcn  Expr=u[1]/(u[1]+u[2])
  pH2O_a_x2 : Outport
  wires:
  Product1/1 -> Sum/1
  mole/sec/1 -> Product1/1, Product/1
  Sum/1 -> RT/Va/1
  RT/Va/1 -> Integrator/1
  Integrator/1 -> pH2O_a_x2/1, Mux/1, Mux1/1
  x6/1 -> mole/sec/1
  Mux/1 -> x1/(x1+x2)/1
  pH2_x1/1 -> Mux/2, Mux1/2
  x1/(x1+x2)/1 -> Product/2
  Product/1 -> Sum/2
  C1/(x1+x2-C2)/1 -> Product1/2
  Mux1/1 -> C1/(x1+x2-C2)/1
  C1/1 -> Mux1/3

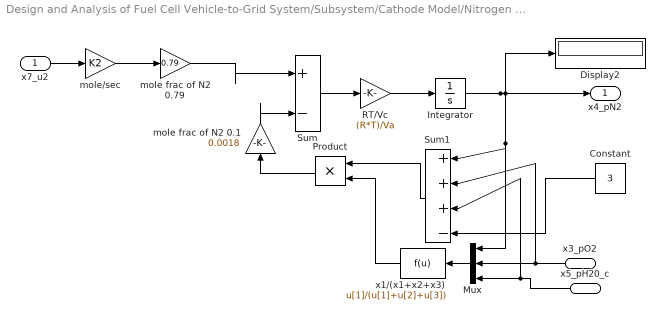
== system Design and Analysis of Fuel Cell Vehicle-to-Grid System/Subsystem/Cathode Model/Nitrogen Model ==
  x7_u2 : Inport
  x3_pO2 : Inport  Port=2
  x5_pH20_c : Inport  Port=3
  Constant : Constant  Value=3
  Display2 : Display
  Integrator : Integrator  InitialCondition=1
  Mux : Mux  Inputs=3
  Product : Product  SaturateOnIntegerOverflow=on  OutDataTypeStr=Inherit: Same as first input
  RT/Vc : Gain  Gain=(R*T)/Va  SaturateOnIntegerOverflow=on  OutDataTypeStr=Inherit: Same as input  ParamDataTypeStr=Inherit: Same as input
  Sum : Sum  Inputs=|+-|  SaturateOnIntegerOverflow=on
  Sum1 : Sum  Inputs=|+++-|  SaturateOnIntegerOverflow=on
  mole frac of N2 0.1 : Gain  Gain=0.0018  SaturateOnIntegerOverflow=on  OutDataTypeStr=Inherit: Same as input  ParamDataTypeStr=Inherit: Same as input
  mole frac of N2 0.79 : Gain  Gain=0.79  SaturateOnIntegerOverflow=on  OutDataTypeStr=Inherit: Same as input  ParamDataTypeStr=Inherit: Same as input
  mole/sec : Gain  Gain=K2  SaturateOnIntegerOverflow=on  OutDataTypeStr=Inherit: Same as input  ParamDataTypeStr=Inherit: Same as input
  x1/(x1+x2+x3) : Fcn  Expr=u[1]/(u[1]+u[2]+u[3])
  x4_pN2 : Outport
  wires:
  mole/sec/1 -> mole frac of N2 0.79/1
  Sum/1 -> RT/Vc/1
  RT/Vc/1 -> Integrator/1
  Integrator/1 -> Display2/1, Mux/1, Sum1/1, x4_pN2/1
  x7_u2/1 -> mole/sec/1
  Mux/1 -> x1/(x1+x2+x3)/1
  x3_pO2/1 -> Mux/2, Sum1/2
  x1/(x1+x2+x3)/1 -> Product/2
  Product/1 -> mole frac of N2 0.1/1
  x5_pH20_c/1 -> Mux/3, Sum1/3
  mole frac of N2 0.79/1 -> Sum/1
  Sum1/1 -> Product/1
  Constant/1 -> Sum1/4
  mole frac of N2 0.1/1 -> Sum/2

== system Design and Analysis of Fuel Cell Vehicle-to-Grid System/Subsystem/Cathode Model/Oxygen Model ==
  x7_u2 : Inport
  x8_Ist : Inport  Port=2
  x4_pN2 : Inport  Port=3
  x5_ pH20_c : Inport  Port=4
  Integrator : Integrator  InitialCondition=1
  Mux : Mux  Inputs=3
  NI/4F : Gain  Gain=N/(4*F)  SaturateOnIntegerOverflow=on  OutDataTypeStr=Inherit: Same as input  ParamDataTypeStr=Inherit: Same as input
  Product : Product  SaturateOnIntegerOverflow=on  OutDataTypeStr=Inherit: Same as first input
  RT/Vc : Gain  Gain=(R*T)/Va  SaturateOnIntegerOverflow=on  OutDataTypeStr=Inherit: Same as input  ParamDataTypeStr=Inherit: Same as input
  Sum : Sum  Inputs=|+--|  SaturateOnIntegerOverflow=on
  Sum1 : Sum  Inputs=|+-|  SaturateOnIntegerOverflow=on
  mole frac of O2 0.21 : Gain  Gain=YO2  SaturateOnIntegerOverflow=on  OutDataTypeStr=Inherit: Same as input  ParamDataTypeStr=Inherit: Same as input
  mole/sec : Gain  Gain=K2  SaturateOnIntegerOverflow=on  OutDataTypeStr=Inherit: Same as input  ParamDataTypeStr=Inherit: Same as input
  x1/(x1+x2) : Fcn  Expr=u[1]/(u[1]+u[2]+u[3])
  x3_pO2 : Outport
  wires:
  mole frac of O2 0.21/1 -> Sum/1
  mole/sec/1 -> mole frac of O2 0.21/1, Sum1/1
  NI/4F/1 -> Sum/2, Sum1/2
  Sum/1 -> RT/Vc/1
  RT/Vc/1 -> Integrator/1
  Integrator/1 -> x3_pO2/1, Mux/1
  x7_u2/1 -> mole/sec/1
  x8_Ist/1 -> NI/4F/1
  Mux/1 -> x1/(x1+x2)/1
  x4_pN2/1 -> Mux/2
  x1/(x1+x2)/1 -> Product/2
  x5_ pH20_c/1 -> Mux/3
  Product/1 -> Sum/3
  Sum1/1 -> Product/1

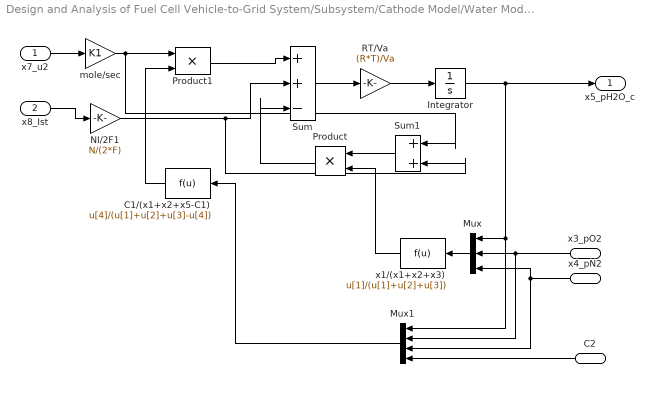
== system Design and Analysis of Fuel Cell Vehicle-to-Grid System/Subsystem/Cathode Model/Water Model  ==
  x7_u2 : Inport
  x8_Ist : Inport  Port=2
  x3_pO2 : Inport  Port=3
  x4_pN2 : Inport  Port=4
  C2 : Inport  Port=5
  C1/(x1+x2+x5-C1) : Fcn  Expr=u[4]/(u[1]+u[2]+u[3]-u[4])
  Integrator : Integrator  InitialCondition=1
  Mux : Mux  Inputs=3
  Mux1 : Mux
  NI/2F1 : Gain  Gain=N/(2*F)  SaturateOnIntegerOverflow=on  OutDataTypeStr=Inherit: Same as input  ParamDataTypeStr=Inherit: Same as input
  Product : Product  SaturateOnIntegerOverflow=on  OutDataTypeStr=Inherit: Same as first input
  Product1 : Product  SaturateOnIntegerOverflow=on  OutDataTypeStr=Inherit: Same as first input
  RT/Va : Gain  Gain=(R*T)/Va  SaturateOnIntegerOverflow=on  OutDataTypeStr=Inherit: Same as input  ParamDataTypeStr=Inherit: Same as input
  Sum : Sum  Inputs=|++-|  SaturateOnIntegerOverflow=on
  Sum1 : Sum  Inputs=|++|  SaturateOnIntegerOverflow=on
  mole/sec : Gain  Gain=K1  SaturateOnIntegerOverflow=on  OutDataTypeStr=Inherit: Same as input  ParamDataTypeStr=Inherit: Same as input
  x1/(x1+x2+x3) : Fcn  Expr=u[1]/(u[1]+u[2]+u[3])
  x5_pH2O_c : Outport
  wires:
  Product1/1 -> Sum/1
  mole/sec/1 -> Product1/1, Sum1/1
  Sum/1 -> RT/Va/1
  RT/Va/1 -> Integrator/1
  Integrator/1 -> x5_pH2O_c/1, Mux/1, Mux1/1
  x7_u2/1 -> mole/sec/1
  Sum1/1 -> Product/1
  Mux/1 -> x1/(x1+x2+x3)/1
  x3_pO2/1 -> Mux/2, Mux1/2
  x1/(x1+x2+x3)/1 -> Product/2
  Product/1 -> Sum/3
  x8_Ist/1 -> NI/2F1/1
  C1/(x1+x2+x5-C1)/1 -> Product1/2
  Mux1/1 -> C1/(x1+x2+x5-C1)/1
  x4_pN2/1 -> Mux/3, Mux1/3
  C2/1 -> Mux1/4
  NI/2F1/1 -> Sum/2, Sum1/2

== system Design and Analysis of Fuel Cell Vehicle-to-Grid System/Subsystem/PI linear Control /Linear PI  v1 ==
  note: PI Curent Regulator
  pO2 : Inport
  Ist : Inport  Port=2
  Constant2 : Constant  Value=3
  Gain1 : Gain  Gain=0  SaturateOnIntegerOverflow=on  OutDataTypeStr=Inherit: Same as input  ParamDataTypeStr=Inherit: Same as input
  Gain2 : Gain  Gain=5  SaturateOnIntegerOverflow=on  OutDataTypeStr=Inherit: Same as input  ParamDataTypeStr=Inherit: Same as input
  Gain3 : Gain  Gain=5  SaturateOnIntegerOverflow=on  OutDataTypeStr=Inherit: Same as input  ParamDataTypeStr=Inherit: Same as input
  Integrator1 : Integrator  LimitOutput=on  UpperSaturationLimit=100  LowerSaturationLimit=-100
  Sum3 : Sum  Inputs=-+  InputSameDT=on  SaturateOnIntegerOverflow=on  OutDataTypeStr=Inherit: Same as first input
  Sum4 : Sum  Inputs=+++  InputSameDT=on  SaturateOnIntegerOverflow=on  OutDataTypeStr=Inherit: Same as first input
  "v2 " : Outport
  wires:
  Gain3/1 -> Sum4/1
  Gain1/1 -> Sum4/3
  Gain2/1 -> Integrator1/1
  Sum3/1 -> Gain3/1, Gain2/1
  Sum4/1 -> "v2 "/1
  Integrator1/1 -> Sum4/2
  Constant2/1 -> Sum3/2
  pO2/1 -> Sum3/1
  Ist/1 -> Gain1/1

== system Design and Analysis of Fuel Cell Vehicle-to-Grid System/Subsystem/PI linear Control /Linear PI  v2 ==
  note: PI Curent Regulator
  pO2 : Inport
  Ist : Inport  Port=2
  Constant2 : Constant  Value=3
  Gain1 : Gain  Gain=0  SaturateOnIntegerOverflow=on  OutDataTypeStr=Inherit: Same as input  ParamDataTypeStr=Inherit: Same as input
  Gain2 : Gain  Gain=50  SaturateOnIntegerOverflow=on  OutDataTypeStr=Inherit: Same as input  ParamDataTypeStr=Inherit: Same as input
  Gain3 : Gain  Gain=50  SaturateOnIntegerOverflow=on  OutDataTypeStr=Inherit: Same as input  ParamDataTypeStr=Inherit: Same as input
  Integrator1 : Integrator  LimitOutput=on  UpperSaturationLimit=1000  LowerSaturationLimit=-1000
  Sum3 : Sum  Inputs=-+  InputSameDT=on  SaturateOnIntegerOverflow=on  OutDataTypeStr=Inherit: Same as first input
  Sum4 : Sum  Inputs=+++  InputSameDT=on  SaturateOnIntegerOverflow=on  OutDataTypeStr=Inherit: Same as first input
  "v2 " : Outport
  wires:
  Gain3/1 -> Sum4/1
  Gain1/1 -> Sum4/3
  Gain2/1 -> Integrator1/1
  Sum3/1 -> Gain3/1, Gain2/1
  Sum4/1 -> "v2 "/1
  Integrator1/1 -> Sum4/2
  Constant2/1 -> Sum3/2
  pO2/1 -> Sum3/1
  Ist/1 -> Gain1/1

== system Design and Analysis of Fuel Cell Vehicle-to-Grid System/Subsystem1/Anode Model/Hydrogen Model ==
  x6 : Inport
  x8 : Inport  Port=2
  pH20_a_x2 : Inport  Port=3
  Display5 : Display
  Integrator : Integrator  InitialCondition=1
  Mux : Mux  Inputs=2
  NI/2F : Gain  Gain=N/(2*F)  SaturateOnIntegerOverflow=on  OutDataTypeStr=Inherit: Same as input  ParamDataTypeStr=Inherit: Same as input
  Product : Product  SaturateOnIntegerOverflow=on  OutDataTypeStr=Inherit: Same as first input
  RT/Va : Gain  Gain=(R*T)/Va  SaturateOnIntegerOverflow=on  OutDataTypeStr=Inherit: Same as input  ParamDataTypeStr=Inherit: Same as input
  Sum : Sum  Inputs=|+--|  SaturateOnIntegerOverflow=on
  Sum1 : Sum  Inputs=|+-|  SaturateOnIntegerOverflow=on
  mole frac of H2 0.99 : Gain  Gain=YH2  SaturateOnIntegerOverflow=on  OutDataTypeStr=Inherit: Same as input  ParamDataTypeStr=Inherit: Same as input
  mole/sec : Gain  Gain=K1  SaturateOnIntegerOverflow=on  OutDataTypeStr=Inherit: Same as input  ParamDataTypeStr=Inherit: Same as input
  x1/(x1+x2) : Fcn  Expr=u[1]/(u[1]+u[2])
  pH2_x1 : Outport
  wires:
  Product/1 -> Sum/3
  x1/(x1+x2)/1 -> Display5/1, Product/2
  pH20_a_x2/1 -> Mux/2
  Mux/1 -> x1/(x1+x2)/1
  Sum1/1 -> Product/1
  x8/1 -> NI/2F/1
  x6/1 -> mole/sec/1
  Integrator/1 -> Mux/1, pH2_x1/1
  RT/Va/1 -> Integrator/1
  Sum/1 -> RT/Va/1
  NI/2F/1 -> Sum1/2, Sum/2
  mole/sec/1 -> Sum1/1, mole frac of H2 0.99/1
  mole frac of H2 0.99/1 -> Sum/1

== system Design and Analysis of Fuel Cell Vehicle-to-Grid System/Subsystem1/Anode Model/Water Model  ==
  x6 : Inport
  pH2_x1 : Inport  Port=2
  C1 : Inport  Port=3
  C1/(x1+x2-C2) : Fcn  Expr=u[3]/(u[1]+u[2]-u[3])
  Integrator : Integrator  InitialCondition=1
  Mux : Mux  Inputs=2
  Mux1 : Mux  Inputs=3
  Product : Product  SaturateOnIntegerOverflow=on  OutDataTypeStr=Inherit: Same as first input
  Product1 : Product  SaturateOnIntegerOverflow=on  OutDataTypeStr=Inherit: Same as first input
  RT/Va : Gain  Gain=(R*T)/Va  SaturateOnIntegerOverflow=on  OutDataTypeStr=Inherit: Same as input  ParamDataTypeStr=Inherit: Same as input
  Sum : Sum  Inputs=|+-|  SaturateOnIntegerOverflow=on
  mole/sec : Gain  Gain=K1  SaturateOnIntegerOverflow=on  OutDataTypeStr=Inherit: Same as input  ParamDataTypeStr=Inherit: Same as input
  x1/(x1+x2) : Fcn  Expr=u[1]/(u[1]+u[2])
  pH2O_a_x2 : Outport
  wires:
  C1/1 -> Mux1/3
  Mux1/1 -> C1/(x1+x2-C2)/1
  C1/(x1+x2-C2)/1 -> Product1/2
  Product/1 -> Sum/2
  x1/(x1+x2)/1 -> Product/2
  pH2_x1/1 -> Mux1/2, Mux/2
  Mux/1 -> x1/(x1+x2)/1
  x6/1 -> mole/sec/1
  Integrator/1 -> Mux1/1, Mux/1, pH2O_a_x2/1
  RT/Va/1 -> Integrator/1
  Sum/1 -> RT/Va/1
  mole/sec/1 -> Product/1, Product1/1
  Product1/1 -> Sum/1

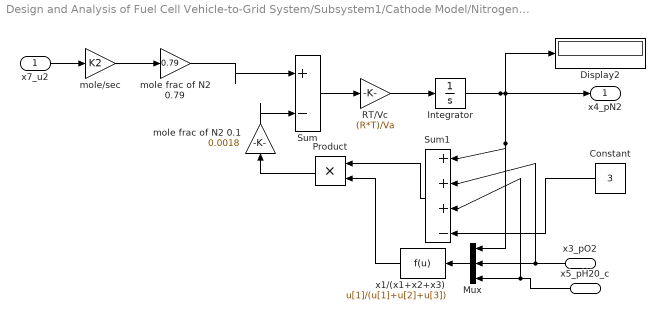
== system Design and Analysis of Fuel Cell Vehicle-to-Grid System/Subsystem1/Cathode Model/Nitrogen Model ==
  x7_u2 : Inport
  x3_pO2 : Inport  Port=2
  x5_pH20_c : Inport  Port=3
  Constant : Constant  Value=3
  Display2 : Display
  Integrator : Integrator  InitialCondition=1
  Mux : Mux  Inputs=3
  Product : Product  SaturateOnIntegerOverflow=on  OutDataTypeStr=Inherit: Same as first input
  RT/Vc : Gain  Gain=(R*T)/Va  SaturateOnIntegerOverflow=on  OutDataTypeStr=Inherit: Same as input  ParamDataTypeStr=Inherit: Same as input
  Sum : Sum  Inputs=|+-|  SaturateOnIntegerOverflow=on
  Sum1 : Sum  Inputs=|+++-|  SaturateOnIntegerOverflow=on
  mole frac of N2 0.1 : Gain  Gain=0.0018  SaturateOnIntegerOverflow=on  OutDataTypeStr=Inherit: Same as input  ParamDataTypeStr=Inherit: Same as input
  mole frac of N2 0.79 : Gain  Gain=0.79  SaturateOnIntegerOverflow=on  OutDataTypeStr=Inherit: Same as input  ParamDataTypeStr=Inherit: Same as input
  mole/sec : Gain  Gain=K2  SaturateOnIntegerOverflow=on  OutDataTypeStr=Inherit: Same as input  ParamDataTypeStr=Inherit: Same as input
  x1/(x1+x2+x3) : Fcn  Expr=u[1]/(u[1]+u[2]+u[3])
  x4_pN2 : Outport
  wires:
  mole frac of N2 0.1/1 -> Sum/2
  Constant/1 -> Sum1/4
  Sum1/1 -> Product/1
  mole frac of N2 0.79/1 -> Sum/1
  x5_pH20_c/1 -> Sum1/3, Mux/3
  Product/1 -> mole frac of N2 0.1/1
  x1/(x1+x2+x3)/1 -> Product/2
  x3_pO2/1 -> Sum1/2, Mux/2
  Mux/1 -> x1/(x1+x2+x3)/1
  x7_u2/1 -> mole/sec/1
  Integrator/1 -> x4_pN2/1, Sum1/1, Mux/1, Display2/1
  RT/Vc/1 -> Integrator/1
  Sum/1 -> RT/Vc/1
  mole/sec/1 -> mole frac of N2 0.79/1

== system Design and Analysis of Fuel Cell Vehicle-to-Grid System/Subsystem1/Cathode Model/Oxygen Model ==
  x7_u2 : Inport
  x8_Ist : Inport  Port=2
  x4_pN2 : Inport  Port=3
  x5_ pH20_c : Inport  Port=4
  Integrator : Integrator  InitialCondition=1
  Mux : Mux  Inputs=3
  NI/4F : Gain  Gain=N/(4*F)  SaturateOnIntegerOverflow=on  OutDataTypeStr=Inherit: Same as input  ParamDataTypeStr=Inherit: Same as input
  Product : Product  SaturateOnIntegerOverflow=on  OutDataTypeStr=Inherit: Same as first input
  RT/Vc : Gain  Gain=(R*T)/Va  SaturateOnIntegerOverflow=on  OutDataTypeStr=Inherit: Same as input  ParamDataTypeStr=Inherit: Same as input
  Sum : Sum  Inputs=|+--|  SaturateOnIntegerOverflow=on
  Sum1 : Sum  Inputs=|+-|  SaturateOnIntegerOverflow=on
  mole frac of O2 0.21 : Gain  Gain=YO2  SaturateOnIntegerOverflow=on  OutDataTypeStr=Inherit: Same as input  ParamDataTypeStr=Inherit: Same as input
  mole/sec : Gain  Gain=K2  SaturateOnIntegerOverflow=on  OutDataTypeStr=Inherit: Same as input  ParamDataTypeStr=Inherit: Same as input
  x1/(x1+x2) : Fcn  Expr=u[1]/(u[1]+u[2]+u[3])
  x3_pO2 : Outport
  wires:
  Sum1/1 -> Product/1
  Product/1 -> Sum/3
  x5_ pH20_c/1 -> Mux/3
  x1/(x1+x2)/1 -> Product/2
  x4_pN2/1 -> Mux/2
  Mux/1 -> x1/(x1+x2)/1
  x8_Ist/1 -> NI/4F/1
  x7_u2/1 -> mole/sec/1
  Integrator/1 -> Mux/1, x3_pO2/1
  RT/Vc/1 -> Integrator/1
  Sum/1 -> RT/Vc/1
  NI/4F/1 -> Sum1/2, Sum/2
  mole/sec/1 -> Sum1/1, mole frac of O2 0.21/1
  mole frac of O2 0.21/1 -> Sum/1

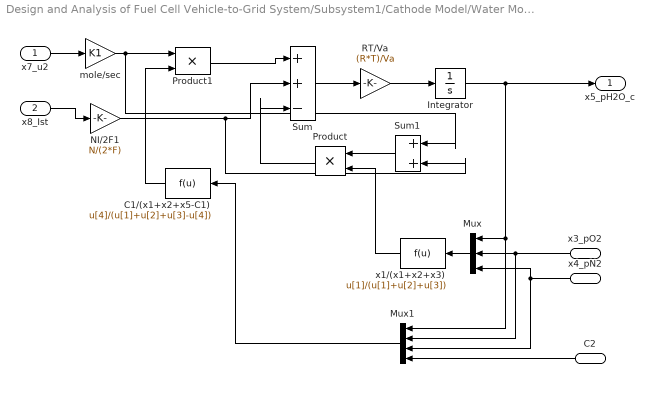
== system Design and Analysis of Fuel Cell Vehicle-to-Grid System/Subsystem1/Cathode Model/Water Model  ==
  x7_u2 : Inport
  x8_Ist : Inport  Port=2
  x3_pO2 : Inport  Port=3
  x4_pN2 : Inport  Port=4
  C2 : Inport  Port=5
  C1/(x1+x2+x5-C1) : Fcn  Expr=u[4]/(u[1]+u[2]+u[3]-u[4])
  Integrator : Integrator  InitialCondition=1
  Mux : Mux  Inputs=3
  Mux1 : Mux
  NI/2F1 : Gain  Gain=N/(2*F)  SaturateOnIntegerOverflow=on  OutDataTypeStr=Inherit: Same as input  ParamDataTypeStr=Inherit: Same as input
  Product : Product  SaturateOnIntegerOverflow=on  OutDataTypeStr=Inherit: Same as first input
  Product1 : Product  SaturateOnIntegerOverflow=on  OutDataTypeStr=Inherit: Same as first input
  RT/Va : Gain  Gain=(R*T)/Va  SaturateOnIntegerOverflow=on  OutDataTypeStr=Inherit: Same as input  ParamDataTypeStr=Inherit: Same as input
  Sum : Sum  Inputs=|++-|  SaturateOnIntegerOverflow=on
  Sum1 : Sum  Inputs=|++|  SaturateOnIntegerOverflow=on
  mole/sec : Gain  Gain=K1  SaturateOnIntegerOverflow=on  OutDataTypeStr=Inherit: Same as input  ParamDataTypeStr=Inherit: Same as input
  x1/(x1+x2+x3) : Fcn  Expr=u[1]/(u[1]+u[2]+u[3])
  x5_pH2O_c : Outport
  wires:
  NI/2F1/1 -> Sum1/2, Sum/2
  C2/1 -> Mux1/4
  x4_pN2/1 -> Mux1/3, Mux/3
  Mux1/1 -> C1/(x1+x2+x5-C1)/1
  C1/(x1+x2+x5-C1)/1 -> Product1/2
  x8_Ist/1 -> NI/2F1/1
  Product/1 -> Sum/3
  x1/(x1+x2+x3)/1 -> Product/2
  x3_pO2/1 -> Mux1/2, Mux/2
  Mux/1 -> x1/(x1+x2+x3)/1
  Sum1/1 -> Product/1
  x7_u2/1 -> mole/sec/1
  Integrator/1 -> Mux1/1, Mux/1, x5_pH2O_c/1
  RT/Va/1 -> Integrator/1
  Sum/1 -> RT/Va/1
  mole/sec/1 -> Sum1/1, Product1/1
  Product1/1 -> Sum/1

== system Design and Analysis of Fuel Cell Vehicle-to-Grid System/Subsystem1/PI linear Control /Linear PI  v1 ==
  note: PI Curent Regulator
  pO2 : Inport
  Ist : Inport  Port=2
  Constant2 : Constant  Value=3
  Gain1 : Gain  Gain=0  SaturateOnIntegerOverflow=on  OutDataTypeStr=Inherit: Same as input  ParamDataTypeStr=Inherit: Same as input
  Gain2 : Gain  Gain=5  SaturateOnIntegerOverflow=on  OutDataTypeStr=Inherit: Same as input  ParamDataTypeStr=Inherit: Same as input
  Gain3 : Gain  Gain=5  SaturateOnIntegerOverflow=on  OutDataTypeStr=Inherit: Same as input  ParamDataTypeStr=Inherit: Same as input
  Integrator1 : Integrator  LimitOutput=on  UpperSaturationLimit=100  LowerSaturationLimit=-100
  Sum3 : Sum  Inputs=-+  InputSameDT=on  SaturateOnIntegerOverflow=on  OutDataTypeStr=Inherit: Same as first input
  Sum4 : Sum  Inputs=+++  InputSameDT=on  SaturateOnIntegerOverflow=on  OutDataTypeStr=Inherit: Same as first input
  "v2 " : Outport
  wires:
  Ist/1 -> Gain1/1
  pO2/1 -> Sum3/1
  Constant2/1 -> Sum3/2
  Integrator1/1 -> Sum4/2
  Sum4/1 -> "v2 "/1
  Sum3/1 -> Gain2/1, Gain3/1
  Gain2/1 -> Integrator1/1
  Gain1/1 -> Sum4/3
  Gain3/1 -> Sum4/1

== system Design and Analysis of Fuel Cell Vehicle-to-Grid System/Subsystem1/PI linear Control /Linear PI  v2 ==
  note: PI Curent Regulator
  pO2 : Inport
  Ist : Inport  Port=2
  Constant2 : Constant  Value=3
  Gain1 : Gain  Gain=0  SaturateOnIntegerOverflow=on  OutDataTypeStr=Inherit: Same as input  ParamDataTypeStr=Inherit: Same as input
  Gain2 : Gain  Gain=50  SaturateOnIntegerOverflow=on  OutDataTypeStr=Inherit: Same as input  ParamDataTypeStr=Inherit: Same as input
  Gain3 : Gain  Gain=50  SaturateOnIntegerOverflow=on  OutDataTypeStr=Inherit: Same as input  ParamDataTypeStr=Inherit: Same as input
  Integrator1 : Integrator  LimitOutput=on  UpperSaturationLimit=1000  LowerSaturationLimit=-1000
  Sum3 : Sum  Inputs=-+  InputSameDT=on  SaturateOnIntegerOverflow=on  OutDataTypeStr=Inherit: Same as first input
  Sum4 : Sum  Inputs=+++  InputSameDT=on  SaturateOnIntegerOverflow=on  OutDataTypeStr=Inherit: Same as first input
  "v2 " : Outport
  wires:
  Ist/1 -> Gain1/1
  pO2/1 -> Sum3/1
  Constant2/1 -> Sum3/2
  Integrator1/1 -> Sum4/2
  Sum4/1 -> "v2 "/1
  Sum3/1 -> Gain2/1, Gain3/1
  Gain2/1 -> Integrator1/1
  Gain1/1 -> Sum4/3
  Gain3/1 -> Sum4/1
